simulink model "trajektorie"  (R2020a)
settings: Solver=VariableStepAuto  StartTime=0.0  StopTime=10.0  RelTol=1e-3
libraries: simulink x1
settings Model: Creator=Ja  LastModifiedBy=Ja

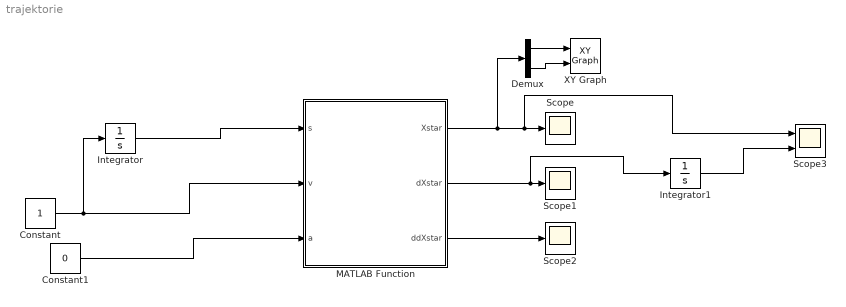
== system trajektorie ==
  Constant : Constant
  Constant1 : Constant  Value=0
  Demux : Demux  Outputs=2
  Integrator : Integrator
  Integrator1 : Integrator
  MATLAB Function : MATLAB Function  TreatAsAtomicUnit=on
  Scope : Scope
  Scope1 : Scope
  Scope2 : Scope
  Scope3 : Scope  NumInputPorts=2
  XY Graph : simulink/Sinks/XY Graph  xmin=0  xmax=5  ymin=-1  ymax=5  st=-1
  wires:
  Constant/1 -> MATLAB Function/2(v), Integrator/1
  Integrator/1 -> MATLAB Function/1(s)
  Constant1/1 -> MATLAB Function/3(a)
  MATLAB Function/1(Xstar) -> Demux/1, Scope3/1, Scope/1
  MATLAB Function/2(dXstar) -> Integrator1/1, Scope1/1
  MATLAB Function/3(ddXstar) -> Scope2/1
  Demux/1 -> XY Graph/1
  Demux/2 -> XY Graph/2
  Integrator1/1 -> Scope3/2

== matlab function trajektorie/MATLAB Function ==
  data: s input; Xstar output size=2; v input; a input; dXstar output size=2; ddXstar output size=2
function [Xstar, dXstar, ddXstar] = MCSstar(s, v, a)

    A = [2 0.5]'
    B = [0 1]'
    C = [2,2.5]'

    r = 0.3
    vmax = 1

    nba = (A - B)/norm(A-B)
    nbc = (C-B)/norm(C-B)
    nbs = (nba+nbc)/norm(nba+nbc)
    K1 = (nba*nba'*nbs-nbs)
    l = r/(sqrt(K1'*K1))
    S = B+nbs*l
    k = nba'*(A-S)
    Pa = A-nba*k
    Pc = B + norm(Pa-B)*nbc
    
%     
%     x_pab = A-k1.*nba
    Pb = B

    helper = (Pa-S)
    fi_pa = atan2(helper(2),helper(1))
    dir = -1
    deltafi = acos(((Pc-S)'*(Pa-S))/r^2)
    
    s1 = norm(Pa-A)
    s2 = norm(Pc-C)
    sk = r*deltafi
    
    if s < s1
        k1 = s
        dk1 = v
        ddk1 = a
        Xstar = A-k1*nba
        dXstar = -dk1*nba
        ddXstar = -ddk1*nba
    elseif s1 <= s &&  s < s1+sk
        Phi = (s-s1)/r
        dPhi = v/r
        ddPhi = a/r
        
        Xstar = r* [cos(fi_pa + dir*Phi); sin(fi_pa + dir*Phi)] + S;
        dXstar = r* [-sin(fi_pa + dir*Phi); cos(fi_pa + dir*Phi)]*dir*dPhi;
        ddXstar = r* [-cos(fi_pa + dir*Phi); -sin(fi_pa + dir*Phi)]*dPhi^2 + r* [-sin(fi_pa + dir*Phi); cos(fi_pa + dir*Phi)]*dir*ddPhi;
    elseif s1+sk < s && s < s1+sk+s2
        k2 = s-s1-sk
        dk2 = v
        ddk2 = a
        
        Xstar = Pc + k2*nbc
        dXstar = dk2*nbc
        ddXstar = ddk2*nbc
    else
%         display('ERROR V TRAJEKTORII')
        Xstar = NaN(2,1)
        dXstar = NaN(2,1)
        ddXstar = NaN(2,1)
    end
   
%     
%     k1 = linspace(0,norm(A-Pa),100)
% 
% 
%     
%     fi = linspace(0,deltafi,100)
%     x_rot = [r*cos(fi_pa+dir*fi);
%              r*sin(fi_pa+dir*fi)]+S
% 
%     k2 = linspace(0,norm(Pc-C),100)
%     x_pbc = Pc + k2.*nbc
% 
% 
% 
%     smax = s1+s2+sk
%     Tmax = smax/vmax
% 
%     T = 100
%     t = linspace(0,Tmax,T)
%     t1 = linspace(0,s1/vmax,T)
%     tk = linspace(s1/vmax,sk/vmax,T)
%     t2 = linspace(sk/vmax,s2/vmax,T)
%     % s = linspace(0,smax,smax/Tmax*10)
%     s = vmax*t
% 
% 
%     k1 = 0+vmax*t
% 
%     k1 = linspace(0,s1,s1/Tmax*T)
%     fi = linspace(0,(sk)/r,(sk)/Tmax*T)
%     k2 = linspace(0,s2,s2/Tmax*T)
% 
%     
%     Xk = [r*cos(fi_pa+dir*fi);r*sin(fi_pa+dir*fi)]+S
%     X2 = Pc+k2.*nbc


end
